simulink model "rTSTemperatureDerate"  (R2024b)
settings: configuration reference "STM32H7_Config" (kept outside this file)
settings Model: DataDictionary=Master_Dictionary.sldd  EnableAccessToBaseWorkspace=off  Creator=torni  LastModifiedBy=William
settings ConfigSetRef: SourceName=STM32H7_Config

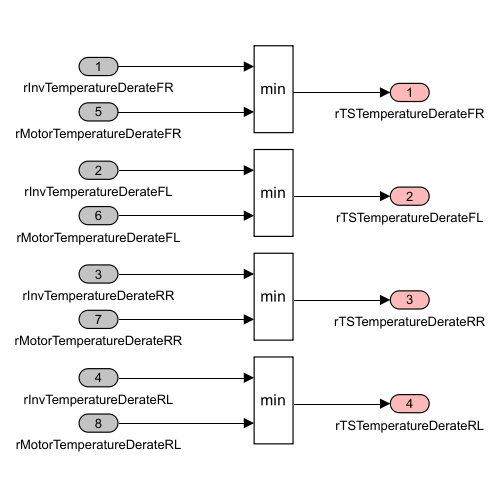
[thumbnail: Simulink's stored preview of the top-level diagram]
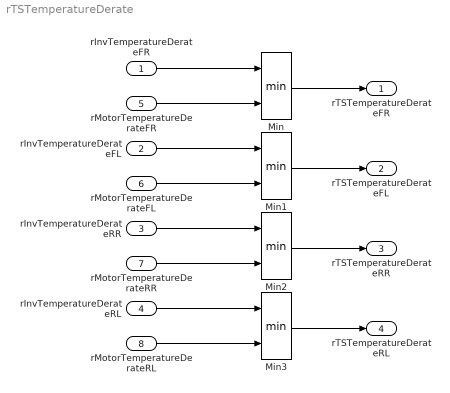
== system rTSTemperatureDerate ==
  rInvTemperatureDerateFR : Inport  OutDataTypeStr=double
  rInvTemperatureDerateFL : Inport  Port=2  OutDataTypeStr=double
  rInvTemperatureDerateRR : Inport  Port=3  OutDataTypeStr=double
  rInvTemperatureDerateRL : Inport  Port=4  OutDataTypeStr=double
  rMotorTemperatureDerateFR : Inport  Port=5  OutDataTypeStr=double
  rMotorTemperatureDerateFL : Inport  Port=6  OutDataTypeStr=double
  rMotorTemperatureDerateRR : Inport  Port=7  OutDataTypeStr=double
  rMotorTemperatureDerateRL : Inport  Port=8  OutDataTypeStr=double
  Min{,1..3} (4 alike) : MinMax  Inputs=2
  rTSTemperatureDerateFR : Outport  OutDataTypeStr=double  VectorParamsAs1DForOutWhenUnconnected=off
  rTSTemperatureDerateFL : Outport  Port=2  OutDataTypeStr=double  VectorParamsAs1DForOutWhenUnconnected=off
  rTSTemperatureDerateRR : Outport  Port=3  OutDataTypeStr=double  VectorParamsAs1DForOutWhenUnconnected=off
  rTSTemperatureDerateRL : Outport  Port=4  OutDataTypeStr=double  VectorParamsAs1DForOutWhenUnconnected=off
  wires:
  Min3/1 -> rTSTemperatureDerateRL/1
  Min2/1 -> rTSTemperatureDerateRR/1
  Min1/1 -> rTSTemperatureDerateFL/1
  Min/1 -> rTSTemperatureDerateFR/1
  rInvTemperatureDerateFR/1 -> Min/1
  rMotorTemperatureDerateFR/1 -> Min/2
  rInvTemperatureDerateFL/1 -> Min1/1
  rMotorTemperatureDerateFL/1 -> Min1/2
  rInvTemperatureDerateRR/1 -> Min2/1
  rMotorTemperatureDerateRR/1 -> Min2/2
  rInvTemperatureDerateRL/1 -> Min3/1
  rMotorTemperatureDerateRL/1 -> Min3/2
